simulink model "quad_new_leg_raibert_strategy_v2"  (R2022b)
settings: Solver=ode15s  StartTime=0.0  StopTime=40  RelTol=1e-3
InitFcn:
  | init_quad_new_leg_raibert_strategy_v2
undefined symbols (not defined in the file): body, ctrl, Extr_Data_LinkEndHole, ground, l1, l2, m1, m2, planner, X, Y, Z
libraries: sm_lib x114, nesl_utility x74, slpidlib x24, simulink x5, Contact_Forces_Lib x4, Parts_Lib x4, sharedtransform x2
(part 7 of 7)

== matlab function quad_new_leg_raibert_strategy_v2/Controller/QuadCtrl ==
  settings: updateMethod=DISCRETE
  data: fl_ang input; tgt_ctrl_fl output; fr_ang input; rl_ang input; rr_ang input; contact_state input; body_R input; sensing_info input; tgt_ctrl_fr output; tgt_ctrl_rl output; tgt_ctrl_rr output; t input; body parameter; planner parameter; mode input; ctrl_state output; debug output; next_state input
function [tgt_ctrl_fl,tgt_ctrl_fr,tgt_ctrl_rl,tgt_ctrl_rr, ctrl_state, debug] = ...
    controller(fl_ang, fr_ang, rl_ang, rr_ang, ...
    contact_state, body_R, sensing_info, t, body, planner, mode, next_state)

% the sample time of the block is set to be 0.0025 (400Hz);
dt = 0.0025;
%unpack sensing_info
body_vx = sensing_info(4);
body_vy = sensing_info(5);

% saggittal angle attempted to be reached by each leg when in turning mode
turn_step = (1-2*(mode==3))*deg2rad(8);

fl_ang_s = fl_ang(1); fl_ang_u = fl_ang(2); fl_ang_k = fl_ang(3);
fr_ang_s = fr_ang(1); fr_ang_u = fr_ang(2); fr_ang_k = fr_ang(3);
rl_ang_s = rl_ang(1); rl_ang_u = rl_ang(2); rl_ang_k = rl_ang(3);
rr_ang_s = rr_ang(1); rr_ang_u = rr_ang(2); rr_ang_k = rr_ang(3);
% forward kinematics
fl_end_effector = forward_kinematics(fl_ang_s, fl_ang_u, fl_ang_k, body); 
rl_end_effector = forward_kinematics(rl_ang_s, rl_ang_u, rl_ang_k, body);
fr_end_effector = forward_kinematics(fr_ang_s, fr_ang_u, fr_ang_k, body);
rr_end_effector = forward_kinematics(rr_ang_s, rr_ang_u, rr_ang_k, body); 

% distance from center of mass to shoulder
fl_offset = [body.shoulder_distance;body.y_length/2+body.shoulder_size/2;0];
fr_offset = [body.shoulder_distance;-body.y_length/2-body.shoulder_size/2;0];
rl_offset = [-body.shoulder_distance;body.y_length/2+body.shoulder_size/2;0];
rr_offset = [-body.shoulder_distance;-body.y_length/2-body.shoulder_size/2;0];

%virtual leg1 fl (front left) rr(rear right) body frame
curr_virtual_leg1 = (fl_end_effector + fl_offset + rr_end_effector + rr_offset)*0.5;
%virtual leg2 fr (front right) rl(rear left) body frame 
curr_virtual_leg2 = (fr_end_effector + fr_offset + rl_end_effector + rl_offset)*0.5;

%decide state and state transition helpers
persistent state;
persistent timer;
persistent timer2;
if isempty(state)
    state = 0;
end
if isempty(timer)
    timer = 0;
end
if isempty(timer2)
    timer2 = 0;
end

% init variables
           % fl fr rl rr
has_u_ctrl = [1 1 1 1];
normal_virtual_leg1 = [0;0;planner.stand_height];
normal_virtual_leg2 = [0;0;planner.stand_height];
move_fl_end_effector = normal_virtual_leg1;
move_rr_end_effector = normal_virtual_leg1;
move_fr_end_effector = normal_virtual_leg2;
move_rl_end_effector = normal_virtual_leg2;
     
% state machine 

if state == 0 % standby state
    % in this state, just do nothing, but use time to make sure that all
    % feet stands on the ground

    if contact_state(1) == 1 && contact_state(2) == 1 && contact_state(3) == 1 && contact_state(4) == 1
        %all foot on ground
        if abs(body_vx) < planner.state0_vel_thres 
            timer = timer + 1;
        else
            timer = 0;
        end
        if timer > planner.state0_trans_thres 
            state = 1;
            timer = 0;
        end
    end
elseif state == 1 % swing whole body to get a inital velocity
    timer2 = timer2 + 1;
    move_theta = planner.state0_swing_ang*sin(2*pi/planner.state0_swing_T*timer2);
    move_leg_Rx = [cos(move_theta) 0 sin(move_theta);
        0 1 0;
        -sin(move_theta) 0 cos(move_theta)];
    tgt_virtual_leg1_b = move_leg_Rx*normal_virtual_leg1;
    tgt_virtual_leg2_b = move_leg_Rx*normal_virtual_leg2;
    move_fl_end_effector = tgt_virtual_leg1_b;
    move_rr_end_effector = tgt_virtual_leg1_b;
    move_fr_end_effector = tgt_virtual_leg2_b;
    move_rl_end_effector = tgt_virtual_leg2_b;
        
    if body_vx > planner.state12_trans_speed
        timer = timer + 1;
    else
        timer = 0;
    end
    if timer > 40  %(keep a velocity larger than 0.2 for 0.1s)
        state = next_state;
        timer = 0;
        timer2 = 0;
    end
    
%%% consider body rotation
% normal_virtual_leg1 = [0;0;planner.stand_height];
% normal_virtual_leg2 = [0;0;planner.stand_height];
% move_fl_end_effector = body_R'*(normal_virtual_leg1+fl_offset)-fl_offset;
% if norm(move_fl_end_effector) > body.max_stretch
%     move_fl_end_effector = move_fl_end_effector/norm(move_fl_end_effector)*body.max_stretch;
% end
% move_rr_end_effector = body_R'*(normal_virtual_leg1+rr_offset)-rr_offset;
% if norm(move_rr_end_effector) > body.max_stretch
%     move_rr_end_effector = move_rr_end_effector/norm(move_rr_end_effector)*body.max_stretch;
% end
% move_fr_end_effector = body_R'*(normal_virtual_leg2+fr_offset)-fr_offset;
% if norm(move_fr_end_effector) > body.max_stretch
%     move_fr_end_effector = move_fr_end_effector/norm(move_fr_end_effector)*body.max_stretch;
% end
% move_rl_end_effector = body_R'*(normal_virtual_leg2+rl_offset)-rl_offset;
% if norm(move_rl_end_effector) > body.max_stretch
%     move_rl_end_effector = move_rl_end_effector/norm(move_rl_end_effector)*body.max_stretch;
% end

elseif state == 2 % stance virtual leg1, swing virtual leg2
    timer2 = timer2 + 1;
    if timer2 > planner.leg_swing_time %(0.5s finish movement)
        timer2 = planner.leg_swing_time;
    end
    % stance leg no u control but need to balance the body
               % fl fr rl rr
    has_u_ctrl = [0 1 1 0];
    t = timer2/planner.leg_swing_time;
%     stance_length_coeff = 0.95+0.05*(timer2/planner.leg_swing_time);
    stance_length_coeff = 0.2*t^2 - 0.2*t + 1;
    tgt_virtual_leg1_b = stance_length_coeff*normal_virtual_leg1;
    move_fl_end_effector = tgt_virtual_leg1_b;
    move_rr_end_effector = tgt_virtual_leg1_b;
    
    
    % swing leg must consider body angle 
%     move_theta = -11/180*pi*(t);
    length_coeff = 0.8*t^2-0.8*t+1;
    % move leg in x direction
    move_theta = get_move_angle(length_coeff*normal_virtual_leg2,body_vx, planner.tgt_body_vx, planner);
    move_leg_Rx = [cos(move_theta) 0 sin(move_theta);
        0 1 0;
        -sin(move_theta) 0 cos(move_theta)];
    tgt_virtual_leg2_b = length_coeff*move_leg_Rx*normal_virtual_leg2;
    % move leg in y direction
    sagittal_angle = get_sagittal_angle(tgt_virtual_leg2_b,body_R, body_vy, planner);
    move_leg_Ry =[1 0 0;
                 0 cos(sagittal_angle) -sin(sagittal_angle);
                 0 sin(sagittal_angle) cos(sagittal_angle)];
    tgt_virtual_leg2_b = move_leg_Ry*tgt_virtual_leg2_b;
    
    
    move_fr_end_effector = body_R'*(tgt_virtual_leg2_b+fr_offset)-fr_offset;
    if norm(move_fr_end_effector) > body.max_stretch
        move_fr_end_effector = move_fr_end_effector/norm(move_fr_end_effector)*body.max_stretch;
    end
    move_rl_end_effector = body_R'*(tgt_virtual_leg2_b+rl_offset)-rl_offset;
    if norm(move_rl_end_effector) > body.max_stretch
        move_rl_end_effector = move_rl_end_effector/norm(move_rl_end_effector)*body.max_stretch;
    end
    
    % state transition
%     if timer2 == planner.leg_swing_time
    if timer2 > 0.5*planner.leg_swing_time && contact_state(2) == 1 && contact_state(3) == 1
        timer = timer + 1;
    else
        timer = 0;
    end
    if timer > 5   % to be determined
        state = next_state;
        timer = 0;
        timer2 = 0;
    end
    
elseif state == 3 % swing virtual leg1, stance virtual leg2
    timer2 = timer2 + 1;
    if timer2 > planner.leg_swing_time %(0.5s finish movement)
        timer2 = planner.leg_swing_time;
    end
    % stance leg no u control but need to balance the body
               % fl fr rl rr
    has_u_ctrl = [1 0 0 1];
%     stance_length_coeff = 0.95+0.05*(timer2/planner.leg_swing_time);
    t = timer2/planner.leg_swing_time;
    stance_length_coeff = 0.2*t^2 - 0.2*t + 1;
    tgt_virtual_leg2_b = stance_length_coeff*normal_virtual_leg2;
    move_fr_end_effector = tgt_virtual_leg2_b;
    move_rl_end_effector = tgt_virtual_leg2_b;
    
    % swing leg must consider body angle 
    % theta is a function of forward velocity 
%     move_theta = -11/180*pi*(t);
    length_coeff = 0.8*t^2-0.8*t+1;
    move_theta = get_move_angle(length_coeff*normal_virtual_leg1,body_vx, planner.tgt_body_vx, planner);
    move_leg_Rx = [cos(move_theta) 0 sin(move_theta);
        0 1 0;
        -sin(move_theta) 0 cos(move_theta)];
    tgt_virtual_leg1_b = length_coeff*move_leg_Rx*normal_virtual_leg1;
        % move leg in y direction
    sagittal_angle = get_sagittal_angle(tgt_virtual_leg1_b,body_R, body_vy, planner);
    move_leg_Ry =[1 0 0;
                 0 cos(sagittal_angle) -sin(sagittal_angle);
                 0 sin(sagittal_angle) cos(sagittal_angle)];
    tgt_virtual_leg1_b = move_leg_Ry*tgt_virtual_leg1_b;
    
    move_fl_end_effector = body_R'*(tgt_virtual_leg1_b+fl_offset)-fl_offset;
    if norm(move_fl_end_effector) > body.max_stretch
        move_fl_end_effector = move_fl_end_effector/norm(move_fl_end_effector)*body.max_stretch;
    end
    move_rr_end_effector = body_R'*(tgt_virtual_leg1_b+rr_offset)-rr_offset;
    if norm(move_rr_end_effector) > body.max_stretch
        move_rr_end_effector = move_rr_end_effector/norm(move_rr_end_effector)*body.max_stretch;
    end
    
    % state transition
%     if timer2 == planner.leg_swing_time
    if timer2 > 0.5*planner.leg_swing_time && contact_state(1) == 1 && contact_state(4) == 1
        timer = timer + 1;
    else
        timer = 0;
    end
    if timer > 5   % to be determined
        state = next_state;
        timer = 0;
        timer2 = 0;
    end
%------------------------------------------------------------------------------------------------------
elseif state == 4 % rotation fl
    timer2 = timer2 + 1;
    if timer2 > planner.leg_swing_time %(0.5s finish movement)
        timer2 = planner.leg_swing_time;
    end
    % stance leg no u control but need to balance the body
               % fl fr rl rr
    has_u_ctrl = [1 0 0 1];
%     stance_length_coeff = 0.95+0.05*(timer2/planner.leg_swing_time);
    t = timer2/planner.leg_swing_time;
    stance_length_coeff = 0.2*t^2 - 0.2*t + 1;
    tgt_virtual_leg2_b = stance_length_coeff*normal_virtual_leg2;
    move_fr_end_effector = tgt_virtual_leg2_b;
    move_rl_end_effector = tgt_virtual_leg2_b;
    
    % swing leg must consider body angle 
    % theta is a function of forward velocity 
%     move_theta = -11/180*pi*(t);
    length_coeff = 0.8*t^2-0.8*t+1;
    %move_theta = get_move_angle(length_coeff*normal_virtual_leg1,body_vx, planner.tgt_body_vx, planner);
    move_theta = planner.state0_swing_ang*sin(2*pi/planner.state0_swing_T*timer2);
    move_leg_Rx = [cos(move_theta) 0 sin(move_theta);
        0 1 0;
        -sin(move_theta) 0 cos(move_theta)];
    tgt_virtual_leg1_b = length_coeff*move_leg_Rx*normal_virtual_leg1;
        % move leg in y direction
    %sagittal_angle = get_sagittal_angle(tgt_virtual_leg1_b,body_R, body_vy, planner);
    sagittal_angle = -turn_step;
    move_leg_Ry =[1 0 0;
                 0 cos(sagittal_angle) -sin(sagittal_angle);
                 0 sin(sagittal_angle) cos(sagittal_angle)];
    tgt_virtual_leg1_b = move_leg_Ry*tgt_virtual_leg1_b;
    
    move_fl_end_effector = body_R'*(tgt_virtual_leg1_b+fl_offset)-fl_offset;
    if norm(move_fl_end_effector) > body.max_stretch
        move_fl_end_effector = move_fl_end_effector/norm(move_fl_end_effector)*body.max_stretch;
    end
    %{
    move_rr_end_effector = body_R'*(tgt_virtual_leg1_b+rr_offset)-rr_offset;
    if norm(move_rr_end_effector) > body.max_stretch
        move_rr_end_effector = move_rr_end_effector/norm(move_rr_end_effector)*body.max_stretch;
    end
    %}
    
    % state transition
%    if timer2 == planner.leg_swing_time
    if timer2 > 0.5*planner.leg_swing_time && contact_state(1) == 1 && contact_state(4) == 1
        timer = timer + 1;
    else
        timer = 0;
    end
    if timer > 5   % to be determined
        state = next_state;
        timer = 0;
        timer2 = 0;
    end
%----------------------------------------------------------------------------------------------------------
elseif state == 5 % rotation fr
    timer2 = timer2 + 1;
    if timer2 > planner.leg_swing_time %(0.5s finish movement)
        timer2 = planner.leg_swing_time;
    end
    % stance leg no u control but need to balance the body
               % fl fr rl rr
    has_u_ctrl = [0 1 1 0];
    t = timer2/planner.leg_swing_time;
%     stance_length_coeff = 0.95+0.05*(timer2/planner.leg_swing_time);
    stance_length_coeff = 0.2*t^2 - 0.2*t + 1;
    tgt_virtual_leg1_b = stance_length_coeff*normal_virtual_leg1;
    move_fl_end_effector = tgt_virtual_leg1_b;
    move_rr_end_effector = tgt_virtual_leg1_b;
    
    
    % swing leg must consider body angle 
%     move_theta = -11/180*pi*(t);
    length_coeff = 0.8*t^2-0.8*t+1;
    % move leg in x direction
    %move_theta = get_move_angle(length_coeff*normal_virtual_leg2,body_vx, planner.tgt_body_vx, planner);
    move_theta = (planner.state0_swing_ang*sin(2*pi/planner.state0_swing_T*timer2));
    move_leg_Rx = [cos(move_theta) 0 sin(move_theta);
        0 1 0;
        -sin(move_theta) 0 cos(move_theta)];
    tgt_virtual_leg2_b = length_coeff*move_leg_Rx*normal_virtual_leg2;
    % move leg in y direction
    %sagittal_angle = get_sagittal_angle(tgt_virtual_leg2_b,body_R, body_vy, planner);
    sagittal_angle = -turn_step;
    move_leg_Ry =[1 0 0;
                 0 cos(sagittal_angle) -sin(sagittal_angle);
                 0 sin(sagittal_angle) cos(sagittal_angle)];
    tgt_virtual_leg2_b = move_leg_Ry*tgt_virtual_leg2_b;
    
    
    move_fr_end_effector = body_R'*(tgt_virtual_leg2_b+fr_offset)-fr_offset;
    if norm(move_fr_end_effector) > body.max_stretch
        move_fr_end_effector = move_fr_end_effector/norm(move_fr_end_effector)*body.max_stretch;
    end
    %{
    move_rl_end_effector = body_R'*(tgt_virtual_leg2_b+rl_offset)-rl_offset;
    if norm(move_rl_end_effector) > body.max_stretch
        move_rl_end_effector = move_rl_end_effector/norm(move_rl_end_effector)*body.max_stretch;
    end
    %}
    
    % state transition
%     if timer2 == planner.leg_swing_time
    if timer2 > 0.5*planner.leg_swing_time && contact_state(2) == 1 && contact_state(3) == 1
        timer = timer + 1;
    else
        timer = 0;
    end
    if timer > 5   % to be determined
        state = next_state;
        timer = 0;
        timer2 = 0;
    end
%-------------------------------------------------------------------------------------------------------
elseif state == 6 % rotation rr
    timer2 = timer2 + 1;
    if timer2 > planner.leg_swing_time %(0.5s finish movement)
        timer2 = planner.leg_swing_time;
    end
    % stance leg no u control but need to balance the body
               % fl fr rl rr
    has_u_ctrl = [1 0 0 1];
%     stance_length_coeff = 0.95+0.05*(timer2/planner.leg_swing_time);
    t = timer2/planner.leg_swing_time;
    stance_length_coeff = 0.2*t^2 - 0.2*t + 1;
    tgt_virtual_leg2_b = stance_length_coeff*normal_virtual_leg2;
    move_fr_end_effector = tgt_virtual_leg2_b;
    move_rl_end_effector = tgt_virtual_leg2_b;
    
    % swing leg must consider body angle 
    % theta is a function of forward velocity 
%     move_theta = -11/180*pi*(t);
    length_coeff = 0.8*t^2-0.8*t+1;
    %move_theta = get_move_angle(length_coeff*normal_virtual_leg1,body_vx, planner.tgt_body_vx, planner);
    move_theta = (planner.state0_swing_ang*sin(2*pi/planner.state0_swing_T*timer2));
    move_leg_Rx = [cos(move_theta) 0 sin(move_theta);
        0 1 0;
        -sin(move_theta) 0 cos(move_theta)];
    tgt_virtual_leg1_b = length_coeff*move_leg_Rx*normal_virtual_leg1;
        % move leg in y direction
    %sagittal_angle = get_sagittal_angle(tgt_virtual_leg1_b,body_R, body_vy, planner);
    sagittal_angle = turn_step;
    move_leg_Ry =[1 0 0;
                 0 cos(sagittal_angle) -sin(sagittal_angle);
                 0 sin(sagittal_angle) cos(sagittal_angle)];
    tgt_virtual_leg1_b = move_leg_Ry*tgt_virtual_leg1_b;
    
    %{
    move_fl_end_effector = body_R'*(tgt_virtual_leg1_b+fl_offset)-fl_offset;
    if norm(move_fl_end_effector) > body.max_stretch
        move_fl_end_effector = move_fl_end_effector/norm(move_fl_end_effector)*body.max_stretch;
    end
    %}
    
    move_rr_end_effector = body_R'*(tgt_virtual_leg1_b+rr_offset)-rr_offset;
    if norm(move_rr_end_effector) > body.max_stretch
        move_rr_end_effector = move_rr_end_effector/norm(move_rr_end_effector)*body.max_stretch;
    end
    
    
    % state transition
%    if timer2 == planner.leg_swing_time
    if timer2 > 0.5*planner.leg_swing_time && contact_state(1) == 1 && contact_state(4) == 1
        timer = timer + 1;
    else
        timer = 0;
    end
    if timer > 5   % to be determined
        state = next_state;
        timer = 0;
        timer2 = 0;
    end
%----------------------------------------------------------------------------------------------------------
elseif state == 7 % rotation rl
    timer2 = timer2 + 1;
    if timer2 > planner.leg_swing_time %(0.5s finish movement)
        timer2 = planner.leg_swing_time;
    end
    % stance leg no u control but need to balance the body
               % fl fr rl rr
    has_u_ctrl = [0 1 1 0];
    t = timer2/planner.leg_swing_time;
%     stance_length_coeff = 0.95+0.05*(timer2/planner.leg_swing_time);
    stance_length_coeff = 0.2*t^2 - 0.2*t + 1;
    tgt_virtual_leg1_b = stance_length_coeff*normal_virtual_leg1;
    move_fl_end_effector = tgt_virtual_leg1_b;
    move_rr_end_effector = tgt_virtual_leg1_b;
    
    
    % swing leg must consider body angle 
%     move_theta = -11/180*pi*(t);
    length_coeff = 0.8*t^2-0.8*t+1;
    % move leg in x direction
    %move_theta = get_move_angle(length_coeff*normal_virtual_leg2,body_vx, planner.tgt_body_vx, planner);
    move_theta = planner.state0_swing_ang*sin(2*pi/planner.state0_swing_T*timer2);
    move_leg_Rx = [cos(move_theta) 0 sin(move_theta);
        0 1 0;
        -sin(move_theta) 0 cos(move_theta)];
    tgt_virtual_leg2_b = length_coeff*move_leg_Rx*normal_virtual_leg2;
    % move leg in y direction
    %sagittal_angle = get_sagittal_angle(tgt_virtual_leg2_b,body_R, body_vy, planner);
    sagittal_angle = turn_step;
    move_leg_Ry =[1 0 0;
                 0 cos(sagittal_angle) -sin(sagittal_angle);
                 0 sin(sagittal_angle) cos(sagittal_angle)];
    tgt_virtual_leg2_b = move_leg_Ry*tgt_virtual_leg2_b;
    
    %{
    move_fr_end_effector = body_R'*(tgt_virtual_leg2_b+fr_offset)-fr_offset;
    if norm(move_fr_end_effector) > body.max_stretch
        move_fr_end_effector = move_fr_end_effector/norm(move_fr_end_effector)*body.max_stretch;
    end
    %}
    move_rl_end_effector = body_R'*(tgt_virtual_leg2_b+rl_offset)-rl_offset;
    if norm(move_rl_end_effector) > body.max_stretch
        move_rl_end_effector = move_rl_end_effector/norm(move_rl_end_effector)*body.max_stretch;
    end
    
    
    % state transition
%     if timer2 == planner.leg_swing_time
    if timer2 > 0.5*planner.leg_swing_time && contact_state(2) == 1 && contact_state(3) == 1
        timer = timer + 1;
    else
        timer = 0;
    end
    if timer > 5   % to be determined
        state = next_state;
        timer = 0;
        timer2 = 0;
    end
%------------------------------------------------------------------------------------------------
elseif state == 8 % stabalisation
    timer2 = timer2 + 1;
    move_theta = planner.state0_swing_ang*sin(2*pi/planner.state0_swing_T*timer2);
    move_leg_Rx = [cos(move_theta) 0 sin(move_theta);
        0 1 0;
        -sin(move_theta) 0 cos(move_theta)];
    tgt_virtual_leg1_b = move_leg_Rx*normal_virtual_leg1;
    tgt_virtual_leg2_b = move_leg_Rx*normal_virtual_leg2;
    move_fl_end_effector = tgt_virtual_leg1_b;
    move_rr_end_effector = tgt_virtual_leg1_b;
    move_fr_end_effector = tgt_virtual_leg2_b;
    move_rl_end_effector = tgt_virtual_leg2_b;
        
    timer = timer + 1;
    if timer > 40  %(keep a velocity larger than 0.2 for 0.1s)
        state = next_state;
        timer = 0;
        timer2 = 0;
    end
end



% delta_ang = planner.swing_ang;
% move_theta1 = delta_ang*sin(2*pi/planner.time_circle*t);
% 
% debug = move_theta1;
% move_leg_y = [cos(move_theta1) 0 sin(move_theta1);
%                             0 1               0;
%              -sin(move_theta1) 0 cos(move_theta1)];
% tgt_virtual_leg1 = move_leg_y*normal_virtual_leg1;
% 
% tgt_virtual_leg2 = move_leg_y'*normal_virtual_leg2;
%          
% 
% move_fl_end_effector = body_R*tgt_virtual_leg1;
% move_rr_end_effector = body_R*tgt_virtual_leg1;
% move_fr_end_effector = body_R*tgt_virtual_leg2;
% move_rl_end_effector = body_R*tgt_virtual_leg2;

%% fl to joint
[inv_s,inv_u,inv_k] = inverse_kinematics(move_fl_end_effector, body);
fl_tgt_ang_s = inv_s; 
fl_tgt_ang_u = inv_u;       
fl_tgt_ang_k = inv_k; 
tgt_ctrl_fl = [fl_tgt_ang_s;fl_tgt_ang_u;fl_tgt_ang_k;has_u_ctrl(1)];

%% fr to joint
[inv_s,inv_u,inv_k] = inverse_kinematics(move_fr_end_effector, body);
fr_tgt_ang_s = inv_s;
fr_tgt_ang_u = inv_u;
fr_tgt_ang_k = inv_k;
tgt_ctrl_fr = [fr_tgt_ang_s;fr_tgt_ang_u;fr_tgt_ang_k;has_u_ctrl(2)];

%% rl to joint
[inv_s,inv_u,inv_k] = inverse_kinematics(move_rl_end_effector, body);
rl_tgt_ang_s = inv_s;
rl_tgt_ang_u = inv_u;
rl_tgt_ang_k = inv_k;
tgt_ctrl_rl = [rl_tgt_ang_s;rl_tgt_ang_u;rl_tgt_ang_k;has_u_ctrl(3)];

%% rr to joint
[inv_s,inv_u,inv_k] = inverse_kinematics(move_rr_end_effector, body);
rr_tgt_ang_s = inv_s;
rr_tgt_ang_u = inv_u;
rr_tgt_ang_k = inv_k; 
tgt_ctrl_rr = [rr_tgt_ang_s;rr_tgt_ang_u;rr_tgt_ang_k;has_u_ctrl(4)];

ctrl_state = state;
debug = timer;

end

function move_angle = get_move_angle(virtual_leg,body_vx, tgt_body_vx, planner)

    distance = body_vx* planner.Ts/2 + planner.Kv*(tgt_body_vx-body_vx);
    
    if distance > 0.5*norm(virtual_leg)
        distance = 0.5*norm(virtual_leg);
    elseif distance < -0.5*norm(virtual_leg)
        distance = -0.5*norm(virtual_leg);
    end
    
    move_angle = asin(distance/norm(virtual_leg));
    if move_angle > 20/180*pi
        move_angle = 20/180*pi;
    elseif move_angle < -20/180*pi
        move_angle = -20/180*pi;
    end
    
end

function move_angle = get_sagittal_angle(virtual_leg,body_R, body_vy, planner)

    distance = body_vy* planner.y_Ts/2 + planner.y_Kv*(0-body_vy);  

    if distance > 0.5*norm(virtual_leg)
        distance = 0.5*norm(virtual_leg);
    elseif distance < -0.5*norm(virtual_leg)
        distance = -0.5*norm(virtual_leg);
    end
    
    move_angle = asin(distance/norm(virtual_leg));
    if move_angle > 20/180*pi
        move_angle = 20/180*pi;
    elseif move_angle < -20/180*pi
        move_angle = -20/180*pi;
    end
    
end

== stateflow chart quad_new_leg_raibert_strategy_v2/Controller/High Level Mode Stateflow ==
  state Stationary
    mode=0;
  state Turning_Right
    mode=2;
  state Walking
    mode=1;
  state Turning_Left
    mode=3;
  (default) -> Stationary : {pos_index = 1}
  Turning_Left -> Stationary : [delta_theta < ang_threshold-0.1]
  Turning_Right -> Stationary : [delta_theta > -ang_threshold+0.1]
  Stationary -> Walking : [~target_reached]
  Walking -> Stationary [order 3] : [target_reached]
      | {pos_index = pos_index + 1}
  Walking -> Turning_Right [order 2] : [delta_theta < -ang_threshold]
  Walking -> Turning_Left [order 1] : [delta_theta > ang_threshold]
  data: pos_index output =0; mode output =0; target_reached input; delta_theta input; ang_threshold local =0.2

== stateflow chart quad_new_leg_raibert_strategy_v2/Controller/State Transitions ==
  state Initilisation
    next_state = 1;
  state Walking_Phase_fr_rl
    next_state = 2;
  state Stationary
    next_state = 8;
  state Turning_Phase_fl
    next_state = 4;
  state Turning_Phase_rr
    next_state = 6;
  state Walking_Phase_fl_rr
    next_state = 3;
  state Turning_Phase_fr
    next_state = 5;
  state Turning_Phase_rl
    next_state = 7;
  (default) -> Initilisation
  Initilisation -> Stationary : [ctrl_state==next_state]
  Stationary -> Turning_Phase_fl [order 2] : [(mode == 2 || mode == 3) && ctrl_state == next_state]
  Turning_Phase_rl -> Turning_Phase_fl [order 2] : [ctrl_state == next_state]
  Stationary -> Walking_Phase_fr_rl [order 1] : [mode == 1 && ctrl_state == next_state]
  Walking_Phase_fl_rr -> Walking_Phase_fr_rl [order 2] : [ctrl_state == next_state]
  Walking_Phase_fr_rl -> (junction 49) [order 1] : [mode ~= 1]
  Turning_Phase_fl -> (junction 49) [order 1] : [mode < 2]
  Walking_Phase_fr_rl -> Walking_Phase_fl_rr [order 2] : [ctrl_state == next_state]
  (junction 49) -> Stationary
  Turning_Phase_fl -> Turning_Phase_rr [order 2] : [ctrl_state == next_state]
  Turning_Phase_rr -> (junction 49) [order 1] : [mode < 2]
  Turning_Phase_rr -> Turning_Phase_fr [order 2] : [ctrl_state == next_state]
  Walking_Phase_fl_rr -> (junction 49) [order 1] : [mode ~= 1]
  Turning_Phase_fr -> (junction 49) [order 1] : [mode < 2]
  Turning_Phase_rl -> (junction 49) [order 1] : [mode < 2]
  Turning_Phase_fr -> Turning_Phase_rl [order 2] : [ctrl_state == next_state]
  data: ctrl_state input =0; mode input =0; next_state output
